simulink model "adder"  (Simulink 5.0)
settings: Solver=FixedStepDiscrete  StartTime=0.0  StopTime=10.0  RelTol=1e-3
settings Model: Creator=sofronis  LastModifiedBy=sofronis  ExtModeAutoUpdateStatusClock=off  AlgebraicLoopMsg=error

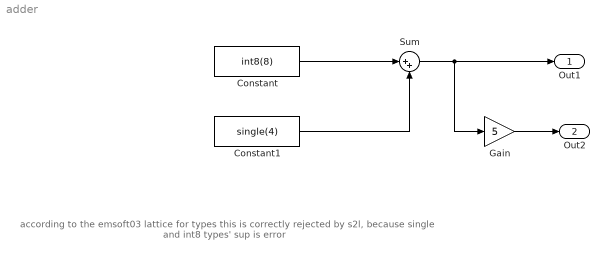
== system adder ==
  note: according to the emsoft03 lattice for
      | types this is correctly rejected by s2l,
      | because single and int8 types' sup is error
  Constant : Constant  Value=int8(8)
  Constant1 : Constant  Value=single(4)
  Gain : Gain  Gain=5  SaturateOnIntegerOverflow=on
  Sum : Sum  Inputs=|++  SaturateOnIntegerOverflow=on
  Out1 : Outport
  Out2 : Outport  Port=2
  wires:
  Constant/1 -> Sum/1
  Constant1/1 -> Sum/2
  Sum/1 -> Out1/1, Gain/1
  Gain/1 -> Out2/1
